simulink model "lateral_SS_F16_Block"  (Simulink 10.0)
settings: Solver=VariableStepAuto  StartTime=0.0  StopTime=200  MaxStep=0.001  RelTol=1e-3
values from neighbouring files (symbols this model uses):
  A = A_hi    [augumentedF16.m]    (also in my_runLINF16sim.m = A_lo; runLINF16sim.m = A_lo)
  B = B_hi    [augumentedF16.m]    (also in my_runLINF16sim.m = B_lo; runLINF16sim.m = B_lo)
  C = eye(18)    [augumentedF16.m]    (also in my_runLINF16sim.m = C_lo; runLINF16sim.m = C_lo)
  D = D_hi    [augumentedF16.m]    (also in my_runLINF16sim.m = D_lo; runLINF16sim.m = D_lo)
  DisAil_1 = AileronDis    (= 0.01)    [augumentedF16.m]    (also in my_runF16Sim.m = 0; my_runLINF16sim.m = 0; runF16Sim.m = 0; runLINF16sim.m = 0)
  DisAil_2 = -2*AileronDis    (= -0.02)    [augumentedF16.m]    (also in my_runF16Sim.m = 0; my_runLINF16sim.m = 0; runF16Sim.m = 0; runLINF16sim.m = 0)
  DisAil_3 = AileronDis    (= 0.01)    [augumentedF16.m]    (also in my_runF16Sim.m = 0; my_runLINF16sim.m = 0; runF16Sim.m = 0; runLINF16sim.m = 0)
  DisEle_1 = ElevatorDis    (= 0.2)    [augumentedF16.m]    (also in my_runF16Sim.m = 0; my_runLINF16sim.m = 0; runF16Sim.m = 0; runLINF16sim.m = 0)
  DisEle_2 = -2*ElevatorDis    (= -0.4)    [augumentedF16.m]    (also in my_runF16Sim.m = 0; my_runLINF16sim.m = 0; runF16Sim.m = 0; runLINF16sim.m = 0)
  DisEle_3 = ElevatorDis    (= 0.2)    [augumentedF16.m]    (also in my_runF16Sim.m = 0; my_runLINF16sim.m = 0; runF16Sim.m = 0; runLINF16sim.m = 0)
  DisRud_1 = RudderDis    (= 0.01)    [augumentedF16.m]    (also in my_runF16Sim.m = 0; my_runLINF16sim.m = 0; runF16Sim.m = 0; runLINF16sim.m = 0)
  DisRud_2 = -2*RudderDis    (= -0.02)    [augumentedF16.m]    (also in my_runF16Sim.m = 0; my_runLINF16sim.m = 0; runF16Sim.m = 0; runLINF16sim.m = 0)
  DisRud_3 = RudderDis    (= 0.01)    [augumentedF16.m]    (also in my_runF16Sim.m = 0; my_runLINF16sim.m = 0; runF16Sim.m = 0; runLINF16sim.m = 0)
  thrust = 5000    [FindF16Dynamics.m]    (also in augumentedF16.m = 0; my_FindF16Dynamics.m; my_runF16Sim.m; my_runLINF16sim.m = 0)
  trim_control = trim_control_hi    [augumentedF16.m]    (also in my_runLINF16sim.m = trim_control_lo; my_trim_F16.m = [xu(2);xu(4);xu(5)]; runLINF16sim.m = trim_control_lo)
  trim_thrust = trim_thrust_hi    [augumentedF16.m]    (also in my_runLINF16sim.m = trim_thrust_lo; my_trim_F16.m = xu(13); runLINF16sim.m = trim_thrust_lo)
undefined symbols (not defined in the file or in its folder): K_lat_phi, K_lat_psi
libraries: simulink_extras x5
settings Model: Creator=asmialek  LastModifiedBy=asmialek
settings DataIOCC: SaveFormat=Dataset
settings OptimizationCC: LifeSpan=auto
settings DebuggingCC: UnderspecifiedInitializationDetection=Simplified  MergeDetectMultiDrivingBlocksExec=error  SFUnexpectedBacktrackingDiag=error  SFNoUnconditionalDefaultTransitionDiag=error  SFExecutionAtInitializationDiag=warning  ArithmeticOperatorsInVariantConditions=error
settings HardwareCC: ProdBitPerPointer=64  ProdBitPerSizeT=64  ProdBitPerPtrDiffT=64  ProdLargestAtomicFloat=Float  ProdIntDivRoundTo=Zero  ProdEndianess=LittleEndian  ProdWordSize=64  ProdHWDeviceType=Intel->x86-64 (Windows64)
settings ModelReferenceCC: PropagateSignalLabelsOutOfModel=on
settings SFSimCC: SimUseLocalCustomCode=on  CustomCodeUndefinedFunction=FilterOut
settings RTWCC: RTWUseLocalCustomCode=on
settings CodeAppCC: StateflowObjectComments=off
settings GRTTargetCC: TargetLangStandard=C99 (ISO)  CombineOutputUpdateFcns=on  GRTInterface=off
settings ConfigComp: CovMetricSettings=dwe  CovHtmlReporting=off  CovSaveCumulativeToWorkspaceVar=off  CovSaveSingleToWorkspaceVar=off

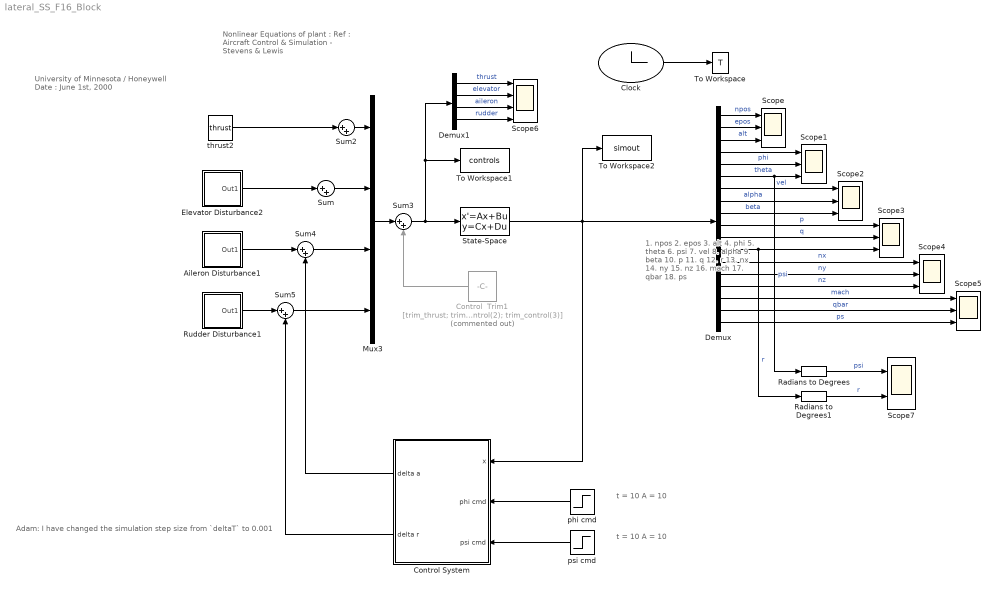
== system lateral_SS_F16_Block ==
  note: Nonlinear Equations of plant :
      | Ref : Aircraft Control & Simulation
      | - Stevens & Lewis
  note: University of Minnesota / Honeywell
      | Date : June 1st, 2000
  note: Adam: I have changed the simulation step size from `deltaT` to 0.001
  note: 1. npos
      | 2. epos
      | 3. alt
      | 4. phi
      | 5. theta
      | 6. psi
      | 7. vel
      | 8. alpha
      | 9. beta
      | 10. p
      | 11. q
      | 12. r
      | 13. nx
      | 14. ny
      | 15. nz
      | 16. mach
      | 17. qbar
      | 18. ps
  note: t = 10
      | A = 10
  note: t = 10
      | A = 10
  Aileron Disturbance1 : Subsystem
  Clock : Clock
      settings: Decimation=50
  Control  Trim1 : Constant  Commented=on  Value=[trim_thrust; trim_control(1); trim_control(2); trim_control(3)]
  Control System : Subsystem
  Demux : Demux  Outputs=18
  Demux1 : Demux
  Elevator Disturbance2 : Subsystem
  Mux3 : Mux
  Radians to Degrees : simulink_extras/Transformations/Radians to Degrees
  Radians to Degrees1 : simulink_extras/Transformations/Radians to Degrees
  Rudder Disturbance1 : Subsystem
  Scope{,1..5} (6 alike) : Scope  NumInputPorts=3
  Scope6 : Scope  NumInputPorts=4
  Scope7 : Scope  NumInputPorts=2
  State-Space : StateSpace  A=A  B=B  C=C  D=D  InitialCondition=0
  Sum{,2..5} (5 alike) : Sum  Inputs=|++
  To Workspace : ToWorkspace  VariableName=T  SampleTime=-1
      settings: Decimation=100
  To Workspace1 : ToWorkspace  VariableName=controls  SampleTime=-1
      settings: Decimation=100
  To Workspace2 : ToWorkspace  VariableName=simout  SampleTime=-1
      settings: Decimation=100
  phi cmd : Step  Time=30  After=10  SampleTime=0  ZeroCross=off
  psi cmd : Step  Time=10  After=10  SampleTime=0  ZeroCross=off
  thrust2 : Constant  Value=thrust  VectorParams1D=off
  wires:
  Demux/3 -> Scope/3  "alt"
  Demux/13 -> Scope4/1  "nx"
  Demux/1 -> Scope/1  "npos"
  Demux/4 -> Scope1/1  "phi"
  Demux/10 -> Scope3/1  "p"
  Demux/6 -> Radians to Degrees/1, Scope1/3  "psi"
  Demux1/4 -> Scope6/4  "rudder"
  Demux/17 -> Scope5/2  "qbar"
  Demux/18 -> Scope5/3  "ps"
  Demux/7 -> Scope2/1  "vel"
  Demux/2 -> Scope/2  "epos"
  Demux1/2 -> Scope6/2  "elevator"
  Demux/15 -> Scope4/3  "nz"
  Demux/11 -> Scope3/2  "q"
  Demux/16 -> Scope5/1  "mach"
  Demux1/1 -> Scope6/1  "thrust"
  Demux1/3 -> Scope6/3  "aileron"
  Demux/5 -> Scope1/2  "theta"
  Demux/12 -> Radians to Degrees1/1, Scope3/3  "r"
  Clock/1 -> To Workspace/1
  Demux/14 -> Scope4/2  "ny"
  Demux/9 -> Scope2/3  "beta"
  Demux/8 -> Scope2/2  "alpha"
  Sum/1 -> Mux3/2
  Elevator Disturbance2/1(Out1) -> Sum/1
  State-Space/1 -> Demux/1, Control System/1(x), To Workspace2/1
  Radians to Degrees/1 -> Scope7/1  "psi"
  Radians to Degrees1/1 -> Scope7/2  "r"
  thrust2/1 -> Sum2/1
  Sum2/1 -> Mux3/1
  Control  Trim1/1 -> Sum3/2
  Mux3/1 -> Sum3/1
  Sum3/1 -> State-Space/1, Demux1/1, To Workspace1/1
  psi cmd/1 -> Control System/3(psi cmd)
  Sum5/1 -> Mux3/4
  Aileron Disturbance1/1(Out1) -> Sum4/1
  Rudder Disturbance1/1(Out1) -> Sum5/1
  Sum4/1 -> Mux3/3
  phi cmd/1 -> Control System/2(phi cmd)
  Control System/2(delta r) -> Sum5/2
  Control System/1(delta a) -> Sum4/2

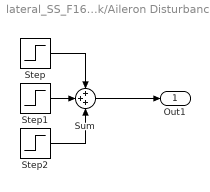
== system lateral_SS_F16_Block/Aileron Disturbance1 ==
  Step : Step  After=DisAil_1  SampleTime=0
  Step1 : Step  Time=3  After=DisAil_2  SampleTime=0
  Step2 : Step  Time=5  After=DisAil_3  SampleTime=0
  Sum : Sum  Inputs=+++  SaturateOnIntegerOverflow=on  InputSameDT=on  OutDataTypeStr=Inherit: Same as first input
  Out1 : Outport
  wires:
  Step1/1 -> Sum/2
  Step/1 -> Sum/1
  Step2/1 -> Sum/3
  Sum/1 -> Out1/1

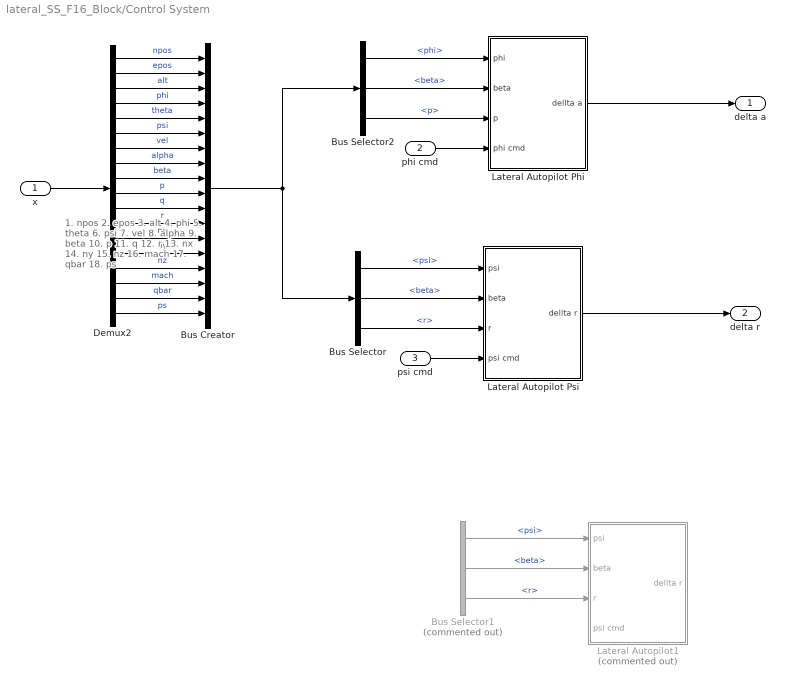
== system lateral_SS_F16_Block/Control System ==
  note: 1. npos
      | 2. epos
      | 3. alt
      | 4. phi
      | 5. theta
      | 6. psi
      | 7. vel
      | 8. alpha
      | 9. beta
      | 10. p
      | 11. q
      | 12. r
      | 13. nx
      | 14. ny
      | 15. nz
      | 16. mach
      | 17. qbar
      | 18. ps
  x : Inport
  phi cmd : Inport  Port=2
  psi cmd : Inport  Port=3
  Bus Creator : BusCreator  Inputs=18
  Bus Selector : BusSelector  OutputSignals=psi,beta,r
  Bus Selector1 : BusSelector  Commented=on  OutputSignals=psi,beta,r
  Bus Selector2 : BusSelector  OutputSignals=phi,beta,p
  Demux2 : Demux  Outputs=18
  Lateral Autopilot Phi : Subsystem
  Lateral Autopilot Psi : Subsystem
  Lateral Autopilot1 : Subsystem  Commented=on
  delta a : Outport
  delta r : Outport  Port=2
  wires:
  x/1 -> Demux2/1
  Demux2/1 -> Bus Creator/1  "npos"
  Demux2/2 -> Bus Creator/2  "epos"
  Demux2/3 -> Bus Creator/3  "alt"
  Demux2/4 -> Bus Creator/4  "phi"
  Demux2/5 -> Bus Creator/5  "theta"
  Demux2/6 -> Bus Creator/6  "psi"
  Demux2/7 -> Bus Creator/7  "vel"
  Demux2/8 -> Bus Creator/8  "alpha"
  Demux2/9 -> Bus Creator/9  "beta"
  Demux2/10 -> Bus Creator/10  "p"
  Demux2/11 -> Bus Creator/11  "q"
  Demux2/12 -> Bus Creator/12  "r"
  Demux2/13 -> Bus Creator/13  "nx"
  Demux2/14 -> Bus Creator/14  "ny"
  Demux2/15 -> Bus Creator/15  "nz"
  Demux2/16 -> Bus Creator/16  "mach"
  Demux2/17 -> Bus Creator/17  "qbar"
  Demux2/18 -> Bus Creator/18  "ps"
  Bus Selector/1 -> Lateral Autopilot Psi/1(psi)  "<psi>"
  Bus Selector/2 -> Lateral Autopilot Psi/2(beta)  "<beta>"
  Bus Selector/3 -> Lateral Autopilot Psi/3(r)  "<r>"
  psi cmd/1 -> Lateral Autopilot Psi/4(" psi cmd")
  Lateral Autopilot Psi/1(dellta r) -> delta r/1
  Bus Selector1/3 -> Lateral Autopilot1/3(r)  "<r>"
  Bus Selector1/1 -> Lateral Autopilot1/1(psi)  "<psi>"
  Bus Selector1/2 -> Lateral Autopilot1/2(beta)  "<beta>"
  Lateral Autopilot Phi/1(dellta a) -> delta a/1
  phi cmd/1 -> Lateral Autopilot Phi/4(" phi cmd")
  Bus Selector2/1 -> Lateral Autopilot Phi/1(phi)  "<phi>"
  Bus Selector2/2 -> Lateral Autopilot Phi/2(beta)  "<beta>"
  Bus Selector2/3 -> Lateral Autopilot Phi/3(p)  "<p>"
  Bus Creator/1 -> Bus Selector/1, Bus Selector2/1

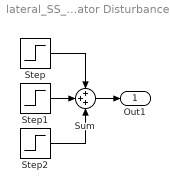
== system lateral_SS_F16_Block/Elevator Disturbance2 ==
  Step : Step  After=DisEle_1  SampleTime=0
  Step1 : Step  Time=3  After=DisEle_2  SampleTime=0
  Step2 : Step  Time=5  After=DisEle_3  SampleTime=0
  Sum : Sum  Inputs=+++  SaturateOnIntegerOverflow=on  InputSameDT=on  OutDataTypeStr=Inherit: Same as first input
  Out1 : Outport
  wires:
  Step1/1 -> Sum/2
  Step/1 -> Sum/1
  Step2/1 -> Sum/3
  Sum/1 -> Out1/1

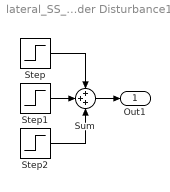
== system lateral_SS_F16_Block/Rudder Disturbance1 ==
  Step : Step  After=DisRud_1  SampleTime=0
  Step1 : Step  Time=1.5  After=DisRud_2  SampleTime=0
  Step2 : Step  Time=2  After=DisRud_3  SampleTime=0
  Sum : Sum  Inputs=+++  SaturateOnIntegerOverflow=on  InputSameDT=on  OutDataTypeStr=Inherit: Same as first input
  Out1 : Outport
  wires:
  Step1/1 -> Sum/2
  Step/1 -> Sum/1
  Step2/1 -> Sum/3
  Sum/1 -> Out1/1

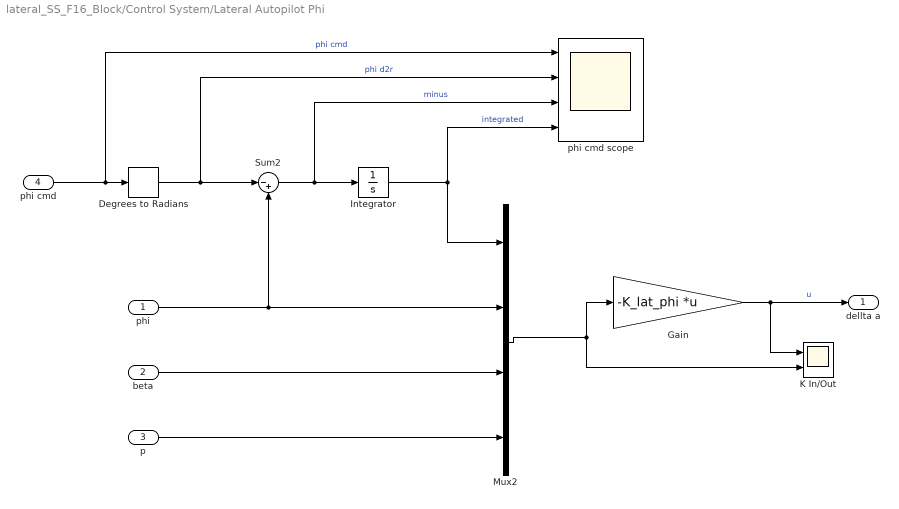
== system lateral_SS_F16_Block/Control System/Lateral Autopilot Phi ==
  phi : Inport
  beta : Inport  Port=2
  p : Inport  Port=3
  " phi cmd" : Inport  Port=4
  Degrees to Radians : simulink_extras/Transformations/Degrees to Radians
  Gain : Gain  Gain=-K_lat_phi  Multiplication=Matrix(K*u)
  Integrator : Integrator
  K In/Out : Scope  NumInputPorts=2
  Mux2 : Mux
  Sum2 : Sum  Inputs=|-+
  phi cmd scope : Scope  NumInputPorts=4
  dellta a : Outport
  wires:
  Mux2/1 -> Gain/1, K In/Out/2
  Gain/1 -> dellta a/1, K In/Out/1  "u"
  Degrees to Radians/1 -> Sum2/1, phi cmd scope/2  "phi d2r"
  " phi cmd"/1 -> Degrees to Radians/1, phi cmd scope/1  "phi cmd"
  Integrator/1 -> phi cmd scope/4, Mux2/1  "integrated"
  Sum2/1 -> phi cmd scope/3, Integrator/1  "minus"
  phi/1 -> Mux2/2, Sum2/2
  p/1 -> Mux2/4
  beta/1 -> Mux2/3

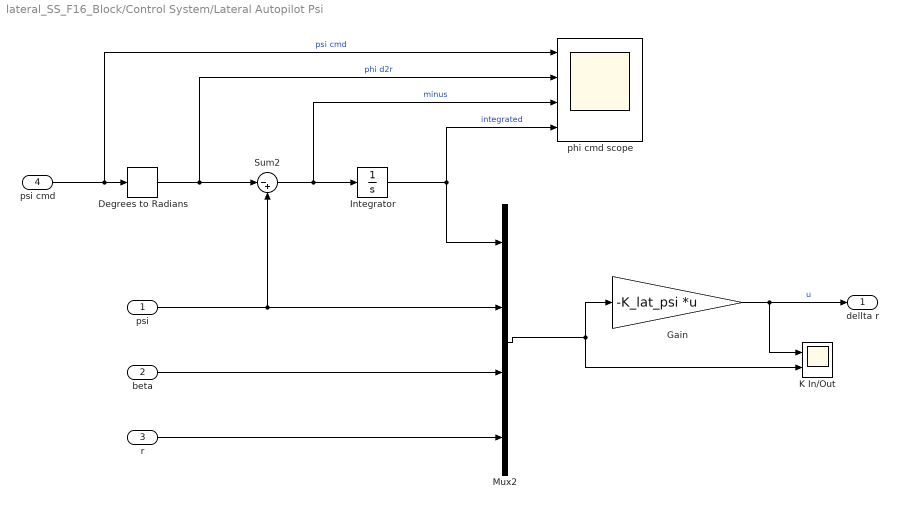
== system lateral_SS_F16_Block/Control System/Lateral Autopilot Psi ==
  psi : Inport
  beta : Inport  Port=2
  r : Inport  Port=3
  " psi cmd" : Inport  Port=4
  Degrees to Radians : simulink_extras/Transformations/Degrees to Radians
  Gain : Gain  Gain=-K_lat_psi  Multiplication=Matrix(K*u)
  Integrator : Integrator
  K In/Out : Scope  NumInputPorts=2
  Mux2 : Mux
  Sum2 : Sum  Inputs=|-+
  phi cmd scope : Scope  NumInputPorts=4
  dellta r : Outport
  wires:
  Mux2/1 -> Gain/1, K In/Out/2
  Gain/1 -> dellta r/1, K In/Out/1  "u"
  Degrees to Radians/1 -> Sum2/1, phi cmd scope/2  "phi d2r"
  " psi cmd"/1 -> Degrees to Radians/1, phi cmd scope/1  "psi cmd"
  Integrator/1 -> phi cmd scope/4, Mux2/1  "integrated"
  Sum2/1 -> phi cmd scope/3, Integrator/1  "minus"
  psi/1 -> Mux2/2, Sum2/2
  r/1 -> Mux2/4
  beta/1 -> Mux2/3

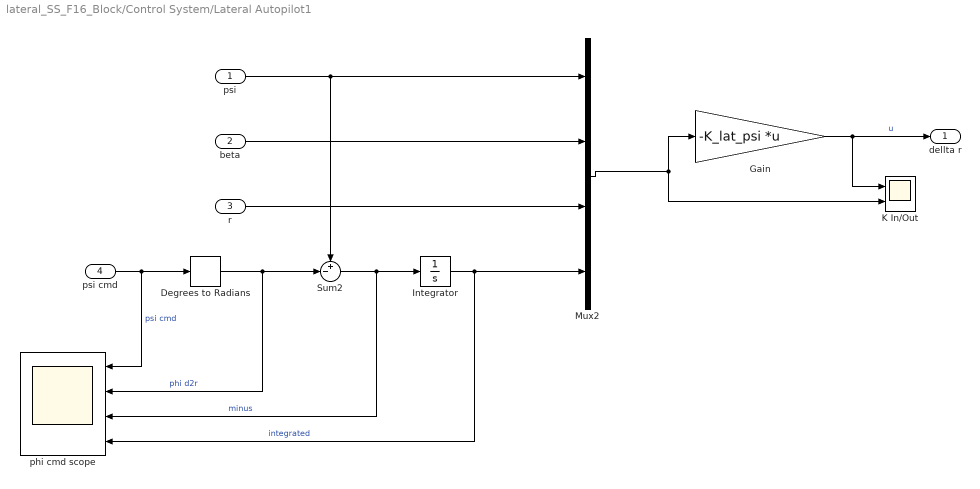
== system lateral_SS_F16_Block/Control System/Lateral Autopilot1 ==
  psi : Inport
  beta : Inport  Port=2
  r : Inport  Port=3
  " psi cmd" : Inport  Port=4
  Degrees to Radians : simulink_extras/Transformations/Degrees to Radians
  Gain : Gain  Gain=-K_lat_psi  Multiplication=Matrix(K*u)
  Integrator : Integrator
  K In/Out : Scope  NumInputPorts=2
  Mux2 : Mux
  Sum2 : Sum  Inputs=+-|
  phi cmd scope : Scope  NumInputPorts=4
  dellta r : Outport
  wires:
  Mux2/1 -> Gain/1, K In/Out/2
  Gain/1 -> dellta r/1, K In/Out/1  "u"
  Integrator/1 -> Mux2/4, phi cmd scope/4  "integrated"
  " psi cmd"/1 -> Degrees to Radians/1, phi cmd scope/1  "psi cmd"
  Degrees to Radians/1 -> Sum2/2, phi cmd scope/2  "phi d2r"
  Sum2/1 -> phi cmd scope/3, Integrator/1  "minus"
  beta/1 -> Mux2/2
  r/1 -> Mux2/3
  psi/1 -> Mux2/1, Sum2/1
